simulink model "Flowchart8"  (Simulink 8.7)
settings: Solver=ode45  StartTime=0.0  StopTime=10.0  RelTol=1e-3
settings Model: Creator=scaife  LastModifiedBy=hamza  ExtModeAutoUpdateStatusClock=off
settings DataIOCC: SignalLoggingSaveFormat=ModelDataLogs  SignalLoggingName=sigsOut
settings OptimizationCC: InitFltsAndDblsToZero=on
settings DebuggingCC: SaveWithParameterizedLinksMsg=none  SignalResolutionControl=TryResolveAllWithWarning  MultiTaskDSMMsg=warning  MultiTaskCondExecSysMsg=none  StrictBusMsg=None
settings HardwareCC: TargetUnknown=on
settings SFSimCC: SimParseCustomCode=off
settings GRTTargetCC: TargetFcnLib=ansi_tfl_tmw.mat  ModelReferenceCompliant=off  GeneratePreprocessorConditionals=Use local settings  CombineOutputUpdateFcns=off  MatFileLogging=off  GRTInterface=on

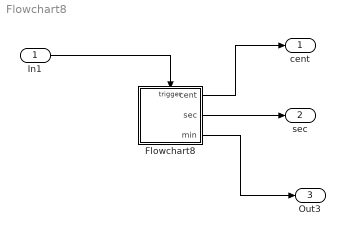
== system Flowchart8 ==
  In1 : Inport
  Flowchart8 : Stateflow chart  TreatAsAtomicUnit=on
  cent : Outport
  sec : Outport  Port=2
  Out3 : Outport  Port=3
  wires:
  In1/1 -> Flowchart8/Trigger
  Flowchart8/1(cent) -> cent/1
  Flowchart8/2(sec) -> sec/1
  Flowchart8/3(min) -> Out3/1

== stateflow chart Flowchart8 ==
  state A
  (default) -> A
  A -> (junction 8) : TIC{cent++}
  (junction 8) -> (junction 10) [order 2]
  (junction 8) -> (junction 9) [order 1] : [cent==2]{cent=0; sec++}
  (junction 9) -> (junction 10) [order 2]
  (junction 9) -> (junction 10) [order 1] : [sec==3]{sec=0; min++}
  data: cent output int32; sec output int32; min output int32
  events: TIC input EITHER_EDGE_EVENT
